simulink library "PowerFlowLib2013amdl"  (Simulink 8.1)
settings: Solver=ode45  StartTime=0.0  StopTime=10.0  RelTol=1e-3
undefined symbols (not defined in the file or in its folder): AirProp, C, F1, Fanmap, Fld1, Fld2, fueltankdata, HydProp, HydraulicLoad, IBFD_exc, L, LoadFluidProps, magnitude, MSSN, n_alghts, PumpProp, pwr_alghts, R_fd_exc, Rcore, Ts, VBFD_exc
libraries: PowerFlowLib x32, simulink x14, powerlib_extras x2, dspstat3 x2
(part 9 of 11)

== system PowerFlowLib2013amdl/Energy & Power Systems/Electrical/Battery/BATTERY/SOC  ==
  INITIAL SOC : Inport
  DCHG CT : Inport  Port=2
  CHG CT : Inport  Port=3
  CHG_DCHG_SIGNAL : Inport  Port=4
  Add1 : Sum  Inputs=+-
  Memory1 : Memory  X0=INITIAL_SOC
  Multiport Switch1 : MultiPortSwitch  DiagnosticForDefault=None
  SOC _ DISCHARGE : Subsystem
  SOC_CHARGE : Subsystem
  Saturation : Saturate  UpperLimit=1  LowerLimit=0
  DYNAMIC SOC : Outport
  NET DCHG CURRENT : Outport  Port=2
  wires:
  Saturation/1 -> Memory1/1, DYNAMIC SOC/1
  Memory1/1 -> Multiport Switch1/4
  Add1/1 -> SOC_CHARGE/2(NET BTRY CT), SOC _ DISCHARGE/2(NET BTRY CT), NET DCHG CURRENT/1
  INITIAL SOC/1 -> SOC_CHARGE/1(INITIAL SOC), SOC _ DISCHARGE/1(INTIAL SOC)
  Multiport Switch1/1 -> Saturation/1
  SOC_CHARGE/1(DYNAMIC SOC) -> Multiport Switch1/3
  DCHG CT/1 -> Add1/1
  CHG CT/1 -> Add1/2
  CHG_DCHG_SIGNAL/1 -> Multiport Switch1/1
  SOC _ DISCHARGE/1(DYNAMIC SOC) -> Multiport Switch1/2

== system PowerFlowLib2013amdl/Energy & Power Systems/Electrical/Converters/Chopper (Averaged)/duty ratio ==
  d(t) : Inport
  Fcn : Fcn  Expr=1-u
  d1(t) : Outport
  d2(t) : Outport  Port=2
  wires:
  d(t)/1 -> d1(t)/1, Fcn/1
  Fcn/1 -> d2(t)/1

== system PowerFlowLib2013amdl/Energy & Power Systems/Electrical/Inverters/ inverter/Three-Phase Full Bridge Inverter CONSTANT FREQUENCY1 ==
  Vdc : Inport
  Inverter current : Inport  Port=2
  Add : Sum
  Constant : Constant  Value=Tr
  Constant1 : Constant  Value=Tf
  Constant2 : Constant  Value=Fsw
  Constant3 : Constant  Value=VCEsat
  No. of IGBT switches : Gain  Gain=Nsw
  "No. of series vol drops " : Gain  Gain=3
  Product : Product  RndMeth=Zero
  Switch Loss : Subsystem
  Total Loss : Outport
  Switching Loss : Outport  Port=2
  Conduction Loss : Outport  Port=3
  wires:
  Constant/1 -> Switch Loss/2(Trise)
  Constant1/1 -> Switch Loss/3(Tfall)
  Inverter current/1 -> Switch Loss/4(Inverter phase current), Product/1
  Switch Loss/1(Switch Loss) -> No. of IGBT switches/1
  Constant2/1 -> Switch Loss/5(Fsw mean)
  Vdc/1 -> Switch Loss/1(Vdc)
  Constant3/1 -> "No. of series vol drops "/1
  "No. of series vol drops "/1 -> Product/2
  Add/1 -> Total Loss/1
  No. of IGBT switches/1 -> Add/1, Switching Loss/1
  Product/1 -> Add/2, Conduction Loss/1

== system PowerFlowLib2013amdl/Energy & Power Systems/Electrical/Inverters/1phs Inverter (2-level) - average/Dot Product ==
  In1 : Inport
  In2 : Inport  Port=2
  S-Function : S-Function  FunctionName=sdotproduct  EnableBusSupport=off
  Out1 : Outport
  wires:
  S-Function/1 -> Out1/1
  In1/1 -> S-Function/1
  In2/1 -> S-Function/2

== system PowerFlowLib2013amdl/Energy & Power Systems/Electrical/Inverters/1phs Inverter (2-level) - average/Dot Product1 ==
  In1 : Inport
  In2 : Inport  Port=2
  S-Function : S-Function  FunctionName=sdotproduct  EnableBusSupport=off
  Out1 : Outport
  wires:
  S-Function/1 -> Out1/1
  In1/1 -> S-Function/1
  In2/1 -> S-Function/2

== system PowerFlowLib2013amdl/Energy & Power Systems/Electrical/Inverters/1phs Inverter (2-level) - switching/2-level PWM ==
  d(t) : Inport
  Data Type Conversion : DataTypeConversion  SaturateOnIntegerOverflow=on  RndMeth=Zero
  Data Type Conversion1 : DataTypeConversion  SaturateOnIntegerOverflow=on  RndMeth=Zero
  Relational Operator : RelationalOperator  Operator=<=  InputSameDT=on
  Relational Operator1 : RelationalOperator  InputSameDT=on
  Tri(t) : Subsystem  mask(Repeating table){rep_seq_t=[0 1/f_s/2 1/f_s], rep_seq_y=[0 1 0]}
      mask prompts: rep_seq_t "Time values:"; rep_seq_y "Output values:"
      mask help: Output a repeating sequence of numbers specified in a table of time-value pairs. Values of time should be monotonically increasing.
      mask init:
      | if (length(rep_seq_t) ~= length(rep_seq_y)),
      |   error('Length of time vector and output vector must be the same.')
      | end
      | dbl_rep_seq_t = double(rep_seq_t);
      | dbl_rep_seq_y = double(rep_seq_y);
      | period = max(dbl_rep_seq_t) - min(dbl_rep_seq_t);
      | period = str2num(sprintf('%0.5g',period));
      | s = round(length(dbl_rep_seq_t)/50);
      | if s > 0
      |   pts = [1:s:length(dbl_rep_seq_t)];
      |   L   = length(pts);
      | else
      |   L   = length(dbl_rep_seq_t);
      |   pts = [1:L];
      | end
      | 
      | disp_seq_t = reshape(dbl_rep_seq_t(pts),L,1);
      | disp_seq_y = reshape(dbl_rep_seq_y(pts),L,1);
      | disp_period = max(disp_seq_t) - min(disp_seq_t);
      | 
      | disp_seq_t  = repmat(disp_seq_t,1,3) + (ones(L,1)*(disp_period*[0,1,2]));
      | disp_seq_t = [ disp_seq_t(:); disp_seq_t(end) ];
      | disp_seq_y = repmat(disp_seq_y,1,3);
      | disp_seq_y = [ disp_seq_y(:); disp_seq_y(1) ];
      mask Help: Repeats cycle given in table. Time values should be monotonically increasing.
      mask Display: plot( disp_seq_t, disp_seq_y )
  q1(t) : Outport
  q2(t) : Outport  Port=2
  wires:
  Relational Operator/1 -> Data Type Conversion/1
  Tri(t)/1(Out1) -> Relational Operator/1, Relational Operator1/1
  Relational Operator1/1 -> Data Type Conversion1/1
  d(t)/1 -> Relational Operator/2, Relational Operator1/2
  Data Type Conversion/1 -> q1(t)/1
  Data Type Conversion1/1 -> q2(t)/1

== system PowerFlowLib2013amdl/Energy & Power Systems/Electrical/Inverters/1phs Inverter (2-level) - switching/Dot Product ==
  In1 : Inport
  In2 : Inport  Port=2
  S-Function : S-Function  FunctionName=sdotproduct  EnableBusSupport=off
  Out1 : Outport
  wires:
  S-Function/1 -> Out1/1
  In1/1 -> S-Function/1
  In2/1 -> S-Function/2

== system PowerFlowLib2013amdl/Energy & Power Systems/Electrical/Inverters/1phs Inverter (2-level) - switching/Dot Product1 ==
  In1 : Inport
  In2 : Inport  Port=2
  S-Function : S-Function  FunctionName=sdotproduct  EnableBusSupport=off
  Out1 : Outport
  wires:
  S-Function/1 -> Out1/1
  In1/1 -> S-Function/1
  In2/1 -> S-Function/2

== system PowerFlowLib2013amdl/Energy & Power Systems/Electrical/Inverters/Inverter (Average)/abc 2 dq ==
  I/P 3 phase : Inport
  angle : Inport  Port=2
  Constant : Constant  Value=2*pi/3
  Constant1 : Constant  Value=2*pi/3
  Demux2 : Demux  Outputs=3
  Gain1 : Gain  Gain=-2/3
  Gain2 : Gain  Gain=2/3
  Mux : Mux  Inputs=2
  Product{,1..5} (6 alike) : Product  RndMeth=Zero
  Sum : Sum  Inputs=|+-
  Sum1 : Sum  Inputs=|+++
  Sum2 : Sum  Inputs=|++
  Sum3 : Sum  Inputs=|+++
  Trigonometric Function : Trigonometry
  Trigonometric Function1 : Trigonometry  Operator=cos
  Trigonometric Function2 : Trigonometry
  Trigonometric Function3 : Trigonometry  Operator=cos
  Trigonometric Function4 : Trigonometry
  Trigonometric Function5 : Trigonometry  Operator=cos
  "O/P 2 phase " : Outport
  wires:
  angle/1 -> Trigonometric Function1/1, Trigonometric Function/1, Sum/1, Sum2/1
  I/P 3 phase/1 -> Demux2/1
  Mux/1 -> "O/P 2 phase "/1
  Trigonometric Function1/1 -> Product2/1
  Demux2/1 -> Product2/2, Product/2
  Constant/1 -> Sum/2
  Constant1/1 -> Sum2/2
  Sum/1 -> Trigonometric Function2/1, Trigonometric Function3/1
  Sum2/1 -> Trigonometric Function4/1, Trigonometric Function5/1
  Demux2/2 -> Product3/2, Product4/2
  Trigonometric Function3/1 -> Product3/1
  Trigonometric Function5/1 -> Product1/1
  Demux2/3 -> Product1/2, Product5/2
  Product2/1 -> Sum1/1
  Product3/1 -> Sum1/2
  Product1/1 -> Sum1/3
  Sum1/1 -> Gain2/1
  Gain2/1 -> Mux/1
  Trigonometric Function/1 -> Product/1
  Trigonometric Function2/1 -> Product4/1
  Trigonometric Function4/1 -> Product5/1
  Product/1 -> Sum3/1
  Product4/1 -> Sum3/2
  Product5/1 -> Sum3/3
  Sum3/1 -> Gain1/1
  Gain1/1 -> Mux/2

== system PowerFlowLib2013amdl/Energy & Power Systems/Electrical/Loads/Constant Current Load/abc to qd0 ==
  note: abc to qd0 reference frame transform (using
      | Krause's notation q = direct axis, d = quadrature axis)
  V_a : Inport
  V_b : Inport  Port=2
  V_c : Inport  Port=3
  Fcn : Fcn  Expr=2/3*(u[1]*cos(0)+u[2]*cos(-2*pi/3)+u[3]*cos(2*pi/3))
  Fcn1 : Fcn  Expr=2/3*(u[1]*sin(0)+u[2]*sin(-2*pi/3)+u[3]*sin(2*pi/3))
  Fcn2 : Fcn  Expr=1/3*(u[1]+u[2]+u[3])
  Mux : Mux  Inputs=3
  V_q : Outport  InitialOutput=0
  V_d : Outport  Port=2  InitialOutput=0
  V_o : Outport  Port=3  InitialOutput=0
  wires:
  Fcn/1 -> V_q/1
  Fcn1/1 -> V_d/1
  Mux/1 -> Fcn/1, Fcn1/1, Fcn2/1
  V_c/1 -> Mux/3
  V_b/1 -> Mux/2
  V_a/1 -> Mux/1
  Fcn2/1 -> V_o/1

== system PowerFlowLib2013amdl/Energy & Power Systems/Electrical/Loads/Constant Power Load/abc to qd0 ==
  note: abc to qd0 reference frame transform (using
      | Krause's notation q = direct axis, d = quadrature axis)
  V_a : Inport
  V_b : Inport  Port=2
  V_c : Inport  Port=3
  Fcn : Fcn  Expr=2/3*(u[1]*cos(0)+u[2]*cos(-2*pi/3)+u[3]*cos(2*pi/3))
  Fcn1 : Fcn  Expr=2/3*(u[1]*sin(0)+u[2]*sin(-2*pi/3)+u[3]*sin(2*pi/3))
  Fcn2 : Fcn  Expr=1/3*(u[1]+u[2]+u[3])
  Mux : Mux  Inputs=3
  V_q : Outport  InitialOutput=0
  V_d : Outport  Port=2  InitialOutput=0
  V_o : Outport  Port=3  InitialOutput=0
  wires:
  Fcn/1 -> V_q/1
  Fcn1/1 -> V_d/1
  Mux/1 -> Fcn/1, Fcn1/1, Fcn2/1
  V_c/1 -> Mux/3
  V_b/1 -> Mux/2
  V_a/1 -> Mux/1
  Fcn2/1 -> V_o/1

== system PowerFlowLib2013amdl/Energy & Power Systems/Electrical/Loads/Enabled_AC_Loadloss/Enabled Subsystem ==
  "Vdq0 " : Inport
  CURRENT BASED LOADS : Subsystem
  IMPEDANCE BASED LOADS : Subsystem
  POWER BASED LOADS : Subsystem
  Sum of Elements : Sum  Inputs=+++
  Idq0 : Outport
  loss : Outport  Port=2
  wires:
  "Vdq0 "/1 -> IMPEDANCE BASED LOADS/1(Vdq0), POWER BASED LOADS/1(Vdq0)
  POWER BASED LOADS/1(Idq0) -> Sum of Elements/1
  CURRENT BASED LOADS/1(Idqo) -> Sum of Elements/2
  Sum of Elements/1 -> Idq0/1
  IMPEDANCE BASED LOADS/1(Idq0) -> Sum of Elements/3
  POWER BASED LOADS/2(loss) -> loss/1

== system PowerFlowLib2013amdl/Energy & Power Systems/Electrical/Loads/Enabled_AC_Loadloss/Enabled Subsystem1 ==
  "Vdq0 " : Inport
  Ext vector : Inport  Port=2
  CURRENT BASED LOADS : Subsystem
  Demux : Demux  Outputs=3
  POWER BASED LOADS : Subsystem
  Sum of Elements : Sum
  Idq0 : Outport
  wires:
  CURRENT BASED LOADS/1(Idqo) -> Sum of Elements/2
  POWER BASED LOADS/1(Idq0) -> Sum of Elements/1
  Sum of Elements/1 -> Idq0/1
  Ext vector/1 -> Demux/1
  "Vdq0 "/1 -> POWER BASED LOADS/1(Vdq0)
  Demux/1 -> POWER BASED LOADS/2(P)
  Demux/2 -> POWER BASED LOADS/3(Q)
  Demux/3 -> CURRENT BASED LOADS/1(Iconst RMS)

== system PowerFlowLib2013amdl/Energy & Power Systems/Electrical/Loss Estimation/Three-Phase ACTIVE RECTIFIER/Switch Loss ==
  Vdc : Inport
  Trise : Inport  Port=2
  Tfall : Inport  Port=3
  Inverter Phae current : Inport  Port=4
  Fsw mean : Inport  Port=5
  Add : Sum
  Divide : Product  Inputs=****
  Gain : Gain  Gain=0.5
  Switching Loss : Outport
  wires:
  Gain/1 -> Divide/2
  Vdc/1 -> Divide/1
  Trise/1 -> Add/1
  Tfall/1 -> Add/2
  Add/1 -> Gain/1
  Inverter Phae current/1 -> Divide/3
  Fsw mean/1 -> Divide/4
  Divide/1 -> Switching Loss/1

== system PowerFlowLib2013amdl/Energy & Power Systems/Electrical/Loss Estimation/Three-Phase ACTIVE RECTIFIER/Switching Frequency ==
  Vdc : Inport
  Source Vol (RMS) : Inport  Port=2
  H-Band : Inport  Port=3
  Lls : Inport  Port=4
  theta : Inport  Port=5
  Add : Sum  Inputs=+-
  Divide : Product  Inputs=**
  Divide1 : Product  Inputs=*/
  Divide2 : Product  Inputs=***
  Gain : Gain  Gain=sqrt(2)
  Gain1 : Gain  Gain=1/(2*pi)
  Gain2 : Gain  Gain=4
  Math Function : Math  Operator=square  SaturateOnIntegerOverflow=on
  Math Function1 : Math  Operator=square  SaturateOnIntegerOverflow=on
  Mean : dspstat3/Mean  run=on  reset_popup=None  InputProcessing=Columns as channels (frame based)  directionMode=Each column  dimension=1  treatSBRowAsCol=on  roiEnable=off  roiType=Rectangles  roiPortion=Entire ROI  roiOutput=Individual statistics for each ROI  roiFlag=off  outputDataTypeStr=Inherit: Same as accumulator  outputLastDataTypeStr=Inherit: Same as accumulator  outputMin=[]  outputMax=[]  roundingMode=Floor  overflowMode=off
  Scope8 : Scope  NumInputPorts=4
      settings: TimeRange=1  YMin=313.1~98040~-1~-5  YMax=313.35~98180~1~5  SaveName=ScopeData9
  Sine : simulink/Lookup Tables/Sine  Formula=sin(2*pi*u)  NumDataPoints=(2^5)+1  OutputWordLength=16
  Zero-Order Hold : ZeroOrderHold  SampleTime=Ts
  Inst. fsw : Outport
  Mean fsw : Outport  Port=2
  wires:
  Vdc/1 -> Divide2/3, Math Function/1, Scope8/1
  Source Vol (RMS)/1 -> Gain/1
  theta/1 -> Gain1/1
  Gain/1 -> Divide/1
  Math Function/1 -> Add/1
  Divide/1 -> Math Function1/1
  Sine/1 -> Divide/2
  Gain1/1 -> Sine/1
  Math Function1/1 -> Add/2
  Add/1 -> Divide1/1, Scope8/2
  H-Band/1 -> Gain2/1
  Gain2/1 -> Divide2/1
  Lls/1 -> Divide2/2
  Divide2/1 -> Divide1/2, Scope8/4
  Divide1/1 -> Zero-Order Hold/1, Inst. fsw/1, Scope8/3
  Mean/1 -> Mean fsw/1
  Zero-Order Hold/1 -> Mean/1

== system PowerFlowLib2013amdl/Energy & Power Systems/Electrical/Loss Estimation/Three-Phase Full Bridge Inverter CONSTANT FREQUENCY/Switch Loss ==
  Vdc : Inport
  Trise : Inport  Port=2
  Tfall : Inport  Port=3
  Inverter phase current : Inport  Port=4
  Fsw mean : Inport  Port=5
  Add : Sum
  Divide : Product  Inputs=****
  Gain : Gain  Gain=0.5
  Switch Loss : Outport
  wires:
  Vdc/1 -> Divide/1
  Trise/1 -> Add/1
  Tfall/1 -> Add/2
  Add/1 -> Gain/1
  Inverter phase current/1 -> Divide/3
  Fsw mean/1 -> Divide/4
  Divide/1 -> Switch Loss/1
  Gain/1 -> Divide/2

== system PowerFlowLib2013amdl/Energy & Power Systems/Electrical/Loss Estimation/Three-Phase Full Bridge Inverter VARIABLE FREQUENCY/Switch Loss ==
  Vdc : Inport
  Trise : Inport  Port=2
  Tfall : Inport  Port=3
  Inverter Phae current : Inport  Port=4
  Fsw mean : Inport  Port=5
  Add : Sum
  Divide : Product  Inputs=****
  Gain : Gain  Gain=0.5
  Switching Loss : Outport
  wires:
  Divide/1 -> Switching Loss/1
  Fsw mean/1 -> Divide/4
  Inverter Phae current/1 -> Divide/3
  Add/1 -> Gain/1
  Tfall/1 -> Add/2
  Trise/1 -> Add/1
  Vdc/1 -> Divide/1
  Gain/1 -> Divide/2

== system PowerFlowLib2013amdl/Energy & Power Systems/Electrical/Loss Estimation/Three-Phase Full Bridge Inverter VARIABLE FREQUENCY/Switching Frequency ==
  Vdc : Inport
  Machine vol (RMS) : Inport  Port=2
  H-Band : Inport  Port=3
  Lls : Inport  Port=4
  theta : Inport  Port=5
  Add : Sum  Inputs=+-
  Divide : Product  Inputs=**
  Divide1 : Product  Inputs=*/
  Divide2 : Product  Inputs=***
  Gain : Gain  Gain=sqrt(2)
  Gain1 : Gain  Gain=1/(2*pi)
  Gain2 : Gain  Gain=4
  Math Function : Math  Operator=square  SaturateOnIntegerOverflow=on
  Math Function1 : Math  Operator=square  SaturateOnIntegerOverflow=on
  Mean : dspstat3/Mean  run=on  reset_popup=None  InputProcessing=Columns as channels (frame based)  directionMode=Each column  dimension=1  treatSBRowAsCol=on  roiEnable=off  roiType=Rectangles  roiPortion=Entire ROI  roiOutput=Individual statistics for each ROI  roiFlag=off  outputDataTypeStr=Inherit: Same as accumulator  outputLastDataTypeStr=Inherit: Same as accumulator  outputMin=[]  outputMax=[]  roundingMode=Floor  overflowMode=off
  Scope8 : Scope  NumInputPorts=4
      settings: TimeRange=1  YMin=313.1~98040~-1~-5  YMax=313.35~98180~1~5  SaveName=ScopeData9
  Sine : simulink/Lookup Tables/Sine  Formula=sin(2*pi*u)  NumDataPoints=(2^5)+1  OutputWordLength=16
  Zero-Order Hold : ZeroOrderHold  SampleTime=Ts
  Inst. fsw : Outport
  Mean fsw : Outport  Port=2
  wires:
  Zero-Order Hold/1 -> Mean/1
  Mean/1 -> Mean fsw/1
  Divide1/1 -> Scope8/3, Inst. fsw/1, Zero-Order Hold/1
  Divide2/1 -> Scope8/4, Divide1/2
  Lls/1 -> Divide2/2
  Gain2/1 -> Divide2/1
  H-Band/1 -> Gain2/1
  Add/1 -> Scope8/2, Divide1/1
  Math Function1/1 -> Add/2
  Gain1/1 -> Sine/1
  Sine/1 -> Divide/2
  Divide/1 -> Math Function1/1
  Math Function/1 -> Add/1
  Gain/1 -> Divide/1
  theta/1 -> Gain1/1
  Machine vol (RMS)/1 -> Gain/1
  Vdc/1 -> Scope8/1, Math Function/1, Divide2/3

== system PowerFlowLib2013amdl/Energy & Power Systems/Electrical/Machines/Induction motor/D-axis block ==
  vds : Inport
  wr*pqr : Inport  Port=2
  Integrator : Integrator
  Integrator1 : Integrator
  Mux : Mux  Inputs=3
  Mux1 : Mux  Inputs=3
  Mux2 : Mux  Inputs=2
  Mux3 : Mux  Inputs=2
  i_ds : Fcn  Expr=1/IM_Xls*(u[2]-u[1])
  pmd : Fcn  Expr=IM_XM*(u[1]/IM_Xls+u[2]/IM_Xplr)
  psi_dr : Fcn  Expr=IM_wb*(-u[2]/IM_wb+IM_rrp/IM_Xplr*(u[1]-u[3]))
  psi_ds : Fcn  Expr=IM_wb*(u[2]+IM_rs/IM_Xls*(u[3]-u[1]))
  pds : Outport
  ids : Outport  Port=2
  pdr : Outport  Port=3
  wires:
  i_ds/1 -> ids/1
  Mux3/1 -> i_ds/1
  wr*pqr/1 -> Mux1/2
  Integrator1/1 -> pdr/1, Mux2/2, Mux1/3
  Integrator/1 -> pds/1, Mux3/2, Mux2/1, Mux/1
  psi_dr/1 -> Integrator1/1
  psi_ds/1 -> Integrator/1
  Mux2/1 -> pmd/1
  Mux1/1 -> psi_dr/1
  pmd/1 -> Mux1/1, Mux3/1, Mux/3
  Mux/1 -> psi_ds/1
  vds/1 -> Mux/2

== system PowerFlowLib2013amdl/Energy & Power Systems/Electrical/Machines/Induction motor/Power Loss Measurement ==
  vqd0s : Inport
  iqd0s : Inport  Port=2
  T_em : Inport  Port=3
  wr_mech : Inport  Port=4
  Gain1 : Gain  Gain=1/Rcore
  Gain2 : Gain  Gain=[3/2 3/2 1]
  Gain3 : Gain  Gain=IM_rs
  Gain4 : Gain  Gain=[3/2 3/2 1].^2
  Gain5 : Gain  Gain=[3/2 3/2 1].^2
  Math Function : Math  Operator=square  SaturateOnIntegerOverflow=on
  Math Function1 : Math  Operator=square  SaturateOnIntegerOverflow=on
  Product : Product  RndMeth=Zero
  Product1 : Product  RndMeth=Zero
  Sum : Sum  Inputs=+
  Sum1 : Sum  Inputs=+-|
  Sum2 : Sum  Inputs=+
  Sum4 : Sum  Inputs=+
  Sum5 : Sum
  P_el : Outport
  P_m : Outport  Port=2
  P_loss : Outport  Port=3
  P_el_loss : Outport  Port=4
  wires:
  Product/1 -> Gain2/1
  vqd0s/1 -> Product/1, Math Function/1
  iqd0s/1 -> Product/2, Math Function1/1
  Gain2/1 -> Sum/1
  Sum/1 -> P_el/1, Sum1/1
  Product1/1 -> P_m/1, Sum1/2
  T_em/1 -> Product1/1
  wr_mech/1 -> Product1/2
  Sum1/1 -> P_loss/1
  Gain1/1 -> Gain5/1
  Gain3/1 -> Gain4/1
  Math Function/1 -> Gain1/1
  Math Function1/1 -> Gain3/1
  Sum2/1 -> Sum5/1
  Sum4/1 -> Sum5/2
  Sum5/1 -> P_el_loss/1
  Gain4/1 -> Sum4/1  "Copper Losses"
  Gain5/1 -> Sum2/1  "Core Loss"

== system PowerFlowLib2013amdl/Energy & Power Systems/Electrical/Machines/Induction motor/Q-axis block ==
  vqs : Inport
  wr*pdr : Inport  Port=2
  Integrator : Integrator
  Integrator1 : Integrator
  Mux : Mux  Inputs=3
  Mux1 : Mux  Inputs=3
  Mux2 : Mux  Inputs=2
  Mux3 : Mux  Inputs=2
  i_qs : Fcn  Expr=1/IM_Xls*(u[2]-u[1])
  pmq : Fcn  Expr=IM_XM*(u[1]/IM_Xls+u[2]/IM_Xplr)
  psi_qr : Fcn  Expr=IM_wb*(u[2]/IM_wb+IM_rrp/IM_Xplr*(u[1]-u[3]))
  psi_qs : Fcn  Expr=IM_wb*(u[2]+IM_rs/IM_Xls*(u[3]-u[1]))
  pqs : Outport
  iqs : Outport  Port=2
  pqr : Outport  Port=3
  wires:
  i_qs/1 -> iqs/1
  Mux3/1 -> i_qs/1
  wr*pdr/1 -> Mux1/2
  Integrator1/1 -> pqr/1, Mux2/2, Mux1/3
  Integrator/1 -> pqs/1, Mux3/2, Mux2/1, Mux/1
  psi_qr/1 -> Integrator1/1
  psi_qs/1 -> Integrator/1
  Mux2/1 -> pmq/1
  Mux1/1 -> psi_qr/1
  pmq/1 -> Mux1/1, Mux3/1, Mux/3
  Mux/1 -> psi_qs/1
  vqs/1 -> Mux/2

== system PowerFlowLib2013amdl/Energy & Power Systems/Electrical/Machines/Permanent Magnet Synchronous Generator1/Generator Power Loss1 ==
  Ploss : Inport
  Tamb : Inport  Port=2
  Gain1 : Gain  Gain=1/mc_exciter
  Heat Trasnfer : Subsystem
  Integrator : Integrator  InitialConditionSource=external
  Sum : Sum  Inputs=|+-
  Ts : Outport
  Pdiss : Outport  Port=2
  wires:
  Gain1/1 -> Integrator/1
  Heat Trasnfer/1(Pdiss) -> Pdiss/1, Sum/2
  Ploss/1 -> Sum/1
  Sum/1 -> Gain1/1
  Integrator/1 -> Heat Trasnfer/2(Ts), Ts/1
  Tamb/1 -> Heat Trasnfer/1(Tamb), Integrator/2

== system PowerFlowLib2013amdl/Energy & Power Systems/Electrical/Machines/Permanent Magnet Synchronous Generator1/Power Loss Measurement ==
  vqd0s : Inport
  iqd0s : Inport  Port=2
  T_em : Inport  Port=3
  wr_mech : Inport  Port=4
  Gain1 : Gain  Gain=1e-10
  Gain2 : Gain  Gain=[3/2 3/2 1]
  Gain3 : Gain  Gain=Rs_pm
  Gain4 : Gain  Gain=[3/2 3/2 1].^2
  Gain5 : Gain  Gain=[3/2 3/2 1].^2
  Math Function : Math  Operator=square  SaturateOnIntegerOverflow=on
  Math Function1 : Math  Operator=square  SaturateOnIntegerOverflow=on
  Product : Product  RndMeth=Zero
  Product1 : Product  RndMeth=Zero
  Sum : Sum  Inputs=+
  Sum1 : Sum  Inputs=-+|
  Sum2 : Sum  Inputs=+
  Sum4 : Sum  Inputs=+
  Sum5 : Sum
  P_el : Outport
  P_m : Outport  Port=2
  P_loss : Outport  Port=3
  P_el_loss : Outport  Port=4
  wires:
  Product/1 -> Gain2/1
  vqd0s/1 -> Product/1, Math Function/1
  iqd0s/1 -> Product/2, Math Function1/1
  Gain2/1 -> Sum/1
  Sum/1 -> P_el/1, Sum1/1
  Product1/1 -> P_m/1, Sum1/2
  T_em/1 -> Product1/1
  wr_mech/1 -> Product1/2
  Sum1/1 -> P_loss/1
  Gain1/1 -> Gain5/1
  Gain3/1 -> Gain4/1
  Math Function/1 -> Gain1/1
  Math Function1/1 -> Gain3/1
  Sum2/1 -> Sum5/1
  Sum4/1 -> Sum5/2
  Sum5/1 -> P_el_loss/1
  Gain4/1 -> Sum4/1  "Copper Losses"
  Gain5/1 -> Sum2/1  "Core Loss"

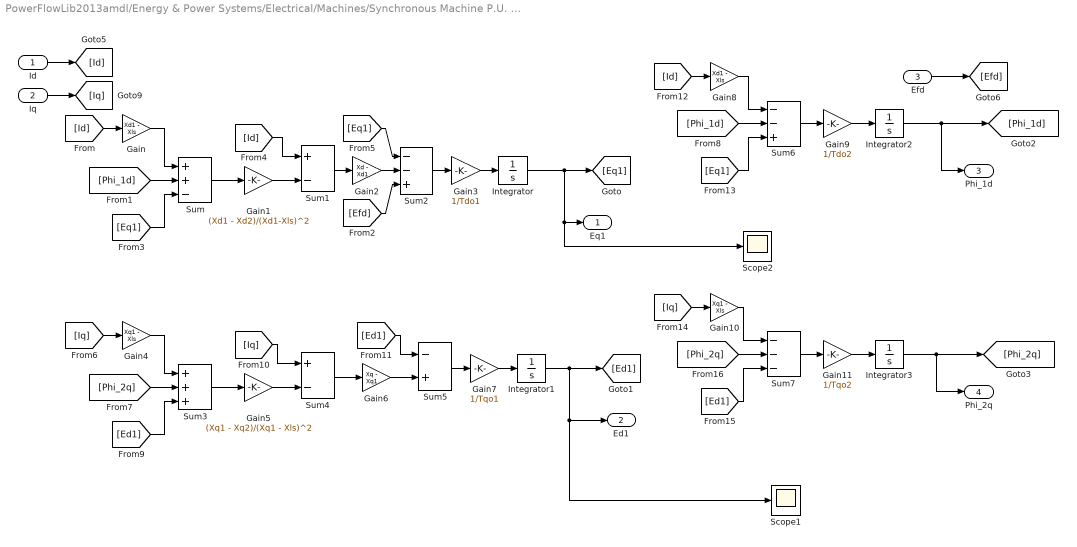
== system PowerFlowLib2013amdl/Energy & Power Systems/Electrical/Machines/Synchronous Machine P.U. dq0/Dynamics ==
  Id : Inport
  Iq : Inport  Port=2
  Efd : Inport  Port=3
  Gain : Gain  Gain=Xd1 - Xls
  Gain1 : Gain  Gain=(Xd1 - Xd2)/(Xd1-Xls)^2
  Gain10 : Gain  Gain=Xq1 - Xls
  Gain11 : Gain  Gain=1/Tqo2
  Gain2 : Gain  Gain=Xd - Xd1
  Gain3 : Gain  Gain=1/Tdo1
  Gain4 : Gain  Gain=Xq1 - Xls
  Gain5 : Gain  Gain=(Xq1 - Xq2)/(Xq1 - Xls)^2
  Gain6 : Gain  Gain=Xq - Xq1
  Gain7 : Gain  Gain=1/Tqo1
  Gain8 : Gain  Gain=Xd1 - Xls
  Gain9 : Gain  Gain=1/Tdo2
  Integrator{,1..3} (4 alike) : Integrator
  Scope1 : Scope
      settings: SaveName=ScopeData6
  Scope2 : Scope
      settings: SaveName=ScopeData7
  Sum : Sum  Inputs=++-
  Sum1 : Sum  Inputs=+-
  Sum2 : Sum  Inputs=--+
  Sum3 : Sum  Inputs=+++
  Sum4 : Sum  Inputs=+-
  Sum5 : Sum  Inputs=-+
  Sum6 : Sum  Inputs=--+
  Sum7 : Sum  Inputs=---
  Eq1 : Outport
  Ed1 : Outport  Port=2
  Phi_1d : Outport  Port=3
  Phi_2q : Outport  Port=4
  wires:
  Efd/1 -> [Efd]
  Iq/1 -> [Iq]
  Id/1 -> [Id]
  Integrator3/1 -> Phi_2q/1, [Phi_2q]
  Gain11/1 -> Integrator3/1
  Sum7/1 -> Gain11/1
  [Ed1] -> Sum7/3
  [Phi_2q] -> Sum7/2
  Gain10/1 -> Sum7/1
  [Iq] -> Gain10/1
  Integrator2/1 -> Phi_1d/1, [Phi_1d]
  Gain9/1 -> Integrator2/1
  Sum6/1 -> Gain9/1
  [Eq1] -> Sum6/3
  [Phi_1d] -> Sum6/2
  Gain8/1 -> Sum6/1
  [Id] -> Gain8/1
  Gain7/1 -> Integrator1/1
  Sum5/1 -> Gain7/1
  Gain6/1 -> Sum5/2
  [Ed1] -> Sum5/1
  Sum4/1 -> Gain6/1
  Gain5/1 -> Sum4/2
  [Iq] -> Sum4/1
  Sum3/1 -> Gain5/1
  [Ed1] -> Sum3/3
  [Phi_2q] -> Sum3/2
  Gain4/1 -> Sum3/1
  [Iq] -> Gain4/1
  Integrator1/1 -> Scope1/1, Ed1/1, [Ed1]
  Gain3/1 -> Integrator/1
  Sum2/1 -> Gain3/1
  [Efd] -> Sum2/3
  Gain2/1 -> Sum2/2
  [Eq1] -> Sum2/1
  Sum1/1 -> Gain2/1
  Gain1/1 -> Sum1/2
  [Id] -> Sum1/1
  Sum/1 -> Gain1/1
  [Eq1] -> Sum/3
  [Phi_1d] -> Sum/2
  Gain/1 -> Sum/1
  [Id] -> Gain/1
  Integrator/1 -> Scope2/1, Eq1/1, [Eq1]

== system PowerFlowLib2013amdl/Energy & Power Systems/Electrical/Machines/Synchronous Machine P.U. dq0/Electromagnetic Torque Output Power ==
  note: Torque from Damper Windings
  note: Torque from Field Winding
  Id : Inport
  Iq : Inport  Port=2
  Eq1 : Inport  Port=3
  Ed1 : Inport  Port=4
  Phi_1d : Inport  Port=5
  Phi_2q : Inport  Port=6
  Gain : Gain  Gain=(Xd2 - Xls)/(Xd1 - Xls)
  Gain1 : Gain  Gain=(Xq2 - Xls)/(Xq1 - Xls)
  Gain2 : Gain  Gain=(Xd1 - Xd2)/(Xd1-Xls)
  Gain3 : Gain  Gain=(Xq1 - Xq2)/(Xq1-Xls)
  Gain4 : Gain  Gain=(Xq2 - Xd2)
  Product{,1..4} (5 alike) : Product  RndMeth=Zero
  Sum : Sum
  Sum1 : Sum  Inputs=+-+
  Sum2 : Sum
  TE : Outport
  wires:
  Sum2/1 -> TE/1
  Sum1/1 -> Sum2/2
  Sum/1 -> Sum2/1
  Gain1/1 -> Sum/2
  Gain/1 -> Sum/1
  Gain4/1 -> Sum1/3
  Gain2/1 -> Sum1/1
  Gain3/1 -> Sum1/2
  Product4/1 -> Gain4/1
  [Iq] -> Product4/2
  [Id] -> Product4/1
  Product3/1 -> Gain3/1
  [Phi_2q] -> Product3/2
  [Id] -> Product3/1
  Product2/1 -> Gain2/1
  [Phi_1d] -> Product2/2
  [Iq] -> Product2/1
  Product1/1 -> Gain1/1
  [Id] -> Product1/2
  [Ed1] -> Product1/1
  Product/1 -> Gain/1
  [Iq] -> Product/2
  [Eq1] -> Product/1
  Iq/1 -> [Iq]
  Phi_2q/1 -> [Phi_2q]
  Phi_1d/1 -> [Phi_1d]
  Ed1/1 -> [Ed1]
  Eq1/1 -> [Eq1]
  Id/1 -> [Id]

== system PowerFlowLib2013amdl/Energy & Power Systems/Electrical/Machines/Synchronous Machine P.U. dq0/Generator Power Loss ==
  Ed : Inport
  Eq : Inport  Port=2
  Id : Inport  Port=3
  Iq : Inport  Port=4
  Te : Inport  Port=5
  w/ws : Inport  Port=6
  Bus Creator : BusCreator  Inputs=6
  Gain1 : Gain  Gain=SB
  Gain2 : Gain  Gain=SB
  Gain3 : Gain  Gain=SB
  Product : Product  RndMeth=Zero
  Product1 : Product  RndMeth=Zero
  Product2 : Product  RndMeth=Zero
  Sum1 : Sum  Inputs=-+
  Sum2 : Sum
  PE : Outport
  PM : Outport  Port=2
  PLOSS : Outport  Port=3
  m : Outport  Port=4
  wires:
  Gain3/1 -> PM/1
  Gain1/1 -> PE/1
  Gain2/1 -> PLOSS/1
  Bus Creator/1 -> m/1
  [nu] -> Bus Creator/6  "nu"
  [Te] -> Bus Creator/5  "Te"
  [Iq] -> Bus Creator/4  "Iq"
  [Eq] -> Bus Creator/3  "Vq"
  [Id] -> Bus Creator/2  "Id"
  [Ed] -> Bus Creator/1  "Vd"
  Sum1/1 -> Gain2/1
  Product2/1 -> Gain3/1, Sum1/2
  Sum2/1 -> Gain1/1, Sum1/1
  Product1/1 -> Sum2/2
  Product/1 -> Sum2/1
  [nu] -> Product2/2
  [Te] -> Product2/1
  [Iq] -> Product1/2
  [Eq] -> Product1/1
  [Id] -> Product/2
  [Ed] -> Product/1
  w/ws/1 -> [nu]
  Te/1 -> [Te]
  Iq/1 -> [Iq]
  Id/1 -> [Id]
  Eq/1 -> [Eq]
  Ed/1 -> [Ed]

== system PowerFlowLib2013amdl/Energy & Power Systems/Electrical/Machines/Synchronous Machine P.U. dq0/Generator Power Loss1 ==
  Ploss : Inport
  Tamb : Inport  Port=2
  Gain1 : Gain  Gain=1/mc_gen
  Heat Trasnfer : Subsystem
  Integrator : Integrator  InitialConditionSource=external
  Sum : Sum  Inputs=|+-
  Ts : Outport
  Pdiss : Outport  Port=2
  wires:
  Gain1/1 -> Integrator/1
  Heat Trasnfer/1(Pdiss) -> Pdiss/1, Sum/2
  Ploss/1 -> Sum/1
  Sum/1 -> Gain1/1
  Integrator/1 -> Heat Trasnfer/2(Ts), Ts/1
  Tamb/1 -> Heat Trasnfer/1(Tamb), Integrator/2

== system PowerFlowLib2013amdl/Energy & Power Systems/Electrical/Machines/Synchronous Machine P.U. dq0/Stator Voltage ==
  Id : Inport
  Iq : Inport  Port=2
  Eq1 : Inport  Port=3
  Ed1 : Inport  Port=4
  Phi_1d : Inport  Port=5
  Phi_2q : Inport  Port=6
  w/ws : Inport  Port=7
  Gain : Gain  Gain=(Xq2 - Xls)/(Xq1 - Xls)
  Gain1 : Gain  Gain=(Xq1 - Xq2)/(Xq1 - Xls)
  Gain2 : Gain  Gain=(Xq2 - Xd2)
  Gain3 : Gain  Gain=(Xd2 - Xls)/(Xd1 - Xls)
  Gain4 : Gain  Gain=(Xd1 - Xd2)/(Xd1 - Xls)
  Gain5 : Gain  Gain=Rs
  Gain6 : Gain  Gain=Xd2+XTL
  Gain7 : Gain  Gain=Rs+RTL
  Gain8 : Gain  Gain=Xd2+XTL
  Product{,1..3} (4 alike) : Product  RndMeth=Zero
  Sum : Sum
  Sum1 : Sum  Inputs=+-+
  Sum2 : Sum  Inputs=--+
  Sum3 : Sum  Inputs=-++
  Ed : Outport
  Eq : Outport  Port=2
  wires:
  Gain7/1 -> Sum2/2
  Product3/1 -> Sum2/1
  Sum2/1 -> Eq/1  "Vq"
  Sum3/1 -> Ed/1  "Vd"
  Product2/1 -> Sum3/3
  Gain2/1 -> Sum1/3
  Product1/1 -> Sum3/2
  Gain8/1 -> Product3/1
  Gain5/1 -> Sum3/1
  Gain6/1 -> Product2/2
  Id/1 -> Gain8/1, Gain5/1
  Product/1 -> Sum2/3
  w/ws/1 -> Product2/1, Product3/2, Product/2, Product1/2
  Sum1/1 -> Product1/1
  Sum/1 -> Product/1
  Gain1/1 -> Sum1/2
  Gain/1 -> Sum1/1
  Gain3/1 -> Sum/1
  Gain4/1 -> Sum/2
  Phi_1d/1 -> Gain4/1
  Eq1/1 -> Gain3/1
  Iq/1 -> Gain2/1, Gain7/1, Gain6/1
  Phi_2q/1 -> Gain1/1
  Ed1/1 -> Gain/1

== system PowerFlowLib2013amdl/Energy & Power Systems/Electrical/Systems/Generation Unit Sync-Sync/Chopper (Averaged) ==
  vin : Inport
  q : Inport  Port=2
  1/R : Gain  Gain=1/(R_fd_exc*VBFD_exc/IBFD_exc)/100/2*3/100  SaturateOnIntegerOverflow=on  OutDataTypeStr=Inherit: Same as input  ParamDataTypeStr=Inherit: Same as input
  Dot Product : DotProduct  InputSameDT=on  OutDataTypeStr=Inherit: Inherit via internal rule
  Dot Product1 : DotProduct  InputSameDT=on  OutDataTypeStr=Inherit: Inherit via internal rule
  Gain2 : Gain  Gain=1000*2/3
  Saturation : Saturate  UpperLimit=1  LowerLimit=0
  iout : Outport
  iin : Outport  Port=2
  wires:
  Dot Product1/1 -> iin/1
  Saturation/1 -> Dot Product1/2, Dot Product/2
  1/R/1 -> Gain2/1
  Dot Product/1 -> 1/R/1
  q/1 -> Saturation/1
  vin/1 -> Dot Product/1
  Gain2/1 -> Dot Product1/1, iout/1

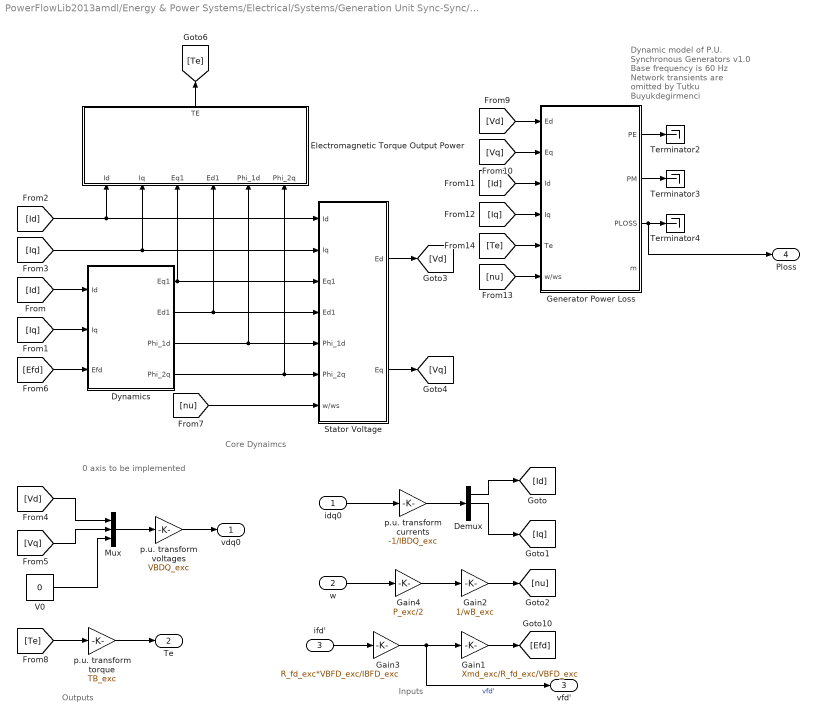
== system PowerFlowLib2013amdl/Energy & Power Systems/Electrical/Systems/Generation Unit Sync-Sync/Exciter ==
  note: 0 axis to be implemented
  note: Inputs
  note: Outputs
  note: Core Dynaimcs
  note: Dynamic model of P.U. Synchronous Generators v1.0
      | Base frequency is 60 Hz
      | Network transients are omitted
      | by Tutku Buyukdegirmenci
  idq0 : Inport
  w : Inport  Port=2
  ifd' : Inport  Port=3
  Demux : Demux  Outputs=3
  Dynamics : Subsystem
  Electromagnetic Torque Output Power : Subsystem
  Gain1 : Gain  Gain=Xmd_exc/R_fd_exc/VBFD_exc
  Gain2 : Gain  Gain=1/wB_exc
  Gain3 : Gain  Gain=R_fd_exc*VBFD_exc/IBFD_exc
  Gain4 : Gain  Gain=P_exc/2
  Generator Power Loss : Subsystem
  Mux : Mux  Inputs=3
  Stator Voltage : Subsystem
  Terminator2 : Terminator
  Terminator3 : Terminator
  Terminator4 : Terminator
  V0 : Constant  Value=0
  p.u. transform currents : Gain  Gain=-1/IBDQ_exc
  p.u. transform torque : Gain  Gain=TB_exc
  p.u. transform voltages : Gain  Gain=VBDQ_exc
  vdq0 : Outport
  Te : Outport  Port=2
  vfd' : Outport  Port=3
  Ploss : Outport  Port=4
  wires:
  Dynamics/1(Eq1) -> Stator Voltage/3(Eq1), Electromagnetic Torque Output Power/3(Eq1)
  Dynamics/2(Ed1) -> Stator Voltage/4(Ed1), Electromagnetic Torque Output Power/4(Ed1)
  Dynamics/3(Phi_1d) -> Stator Voltage/5(Phi_1d), Electromagnetic Torque Output Power/5(Phi_1d)
  Dynamics/4(Phi_2q) -> Stator Voltage/6(Phi_2q), Electromagnetic Torque Output Power/6(Phi_2q)
  Stator Voltage/2(Eq) -> [Vq]
  Stator Voltage/1(Ed) -> [Vd]
  w/1 -> Gain4/1
  Demux/1 -> [Id]
  Demux/2 -> [Iq]
  Gain2/1 -> [nu]
  [Id] -> Dynamics/1(Id)
  [Iq] -> Dynamics/2(Iq)
  [Id] -> Stator Voltage/1(Id), Electromagnetic Torque Output Power/1(Id)
  [Iq] -> Stator Voltage/2(Iq), Electromagnetic Torque Output Power/2(Iq)
  Mux/1 -> p.u. transform voltages/1
  [Vd] -> Mux/1
  [Vq] -> Mux/2
  V0/1 -> Mux/3
  [nu] -> Stator Voltage/7(w/ws)
  Electromagnetic Torque Output Power/1(TE) -> [Te]
  [Te] -> p.u. transform torque/1
  p.u. transform currents/1 -> Demux/1
  p.u. transform torque/1 -> Te/1
  [Vd] -> Generator Power Loss/1(Ed)
  [Vq] -> Generator Power Loss/2(Eq)
  [Id] -> Generator Power Loss/3(Id)
  [Iq] -> Generator Power Loss/4(Iq)
  [nu] -> Generator Power Loss/6(w/ws)
  [Te] -> Generator Power Loss/5(Te)
  Generator Power Loss/1(PE) -> Terminator2/1
  Generator Power Loss/2(PM) -> Terminator3/1
  Generator Power Loss/3(PLOSS) -> Ploss/1, Terminator4/1
  p.u. transform voltages/1 -> vdq0/1
  idq0/1 -> p.u. transform currents/1
  ifd'/1 -> Gain3/1
  Gain1/1 -> [Efd]
  Gain3/1 -> vfd'/1, Gain1/1  "vfd'"
  [Efd] -> Dynamics/3(Efd)
  Gain4/1 -> Gain2/1

== system PowerFlowLib2013amdl/Energy & Power Systems/Electrical/Systems/Generation Unit Sync-Sync/Generator ==
  note: Dynamic model of P.U. Synchronous Generators v1.0
      | Base frequency is 60 Hz
      | Network transients are omitted
      | by Tutku Buyukdegirmenci
  note: Core Dynaimcs
  note: Outputs
  note: Inputs
  note: 0 axis to be implemented
  idq0 : Inport
  w : Inport  Port=2
  ifd' : Inport  Port=3
  Demux : Demux  Outputs=3
  Dynamics : Subsystem
  Electromagnetic Torque Output Power : Subsystem
  Gain1 : Gain  Gain=Xmd/R_fd/VBFD
  Gain2 : Gain  Gain=1/wB
  Gain3 : Gain  Gain=R_fd*VBFD/IBFD
  Gain4 : Gain  Gain=P/2
  Generator Power Loss : Subsystem
  Mux : Mux  Inputs=3
  Stator Voltage : Subsystem
  Terminator2 : Terminator
  Terminator3 : Terminator
  Terminator4 : Terminator
  V0 : Constant  Value=0
  p.u. transform currents : Gain  Gain=-1/IBDQ
  p.u. transform torque : Gain  Gain=TB
  p.u. transform voltages : Gain  Gain=VBDQ
  vdq0 : Outport
  Te : Outport  Port=2
  vfd' : Outport  Port=3
  Ploss : Outport  Port=4
  wires:
  Gain4/1 -> Gain2/1
  [Efd] -> Dynamics/3(Efd)
  Gain3/1 -> vfd'/1, Gain1/1  "vfd'"
  Gain1/1 -> [Efd]
  ifd'/1 -> Gain3/1
  idq0/1 -> p.u. transform currents/1
  p.u. transform voltages/1 -> vdq0/1
  Generator Power Loss/3(PLOSS) -> Ploss/1, Terminator4/1
  Generator Power Loss/2(PM) -> Terminator3/1
  Generator Power Loss/1(PE) -> Terminator2/1
  [Te] -> Generator Power Loss/5(Te)
  [nu] -> Generator Power Loss/6(w/ws)
  [Iq] -> Generator Power Loss/4(Iq)
  [Id] -> Generator Power Loss/3(Id)
  [Vq] -> Generator Power Loss/2(Eq)
  [Vd] -> Generator Power Loss/1(Ed)
  p.u. transform torque/1 -> Te/1
  p.u. transform currents/1 -> Demux/1
  [Te] -> p.u. transform torque/1
  Electromagnetic Torque Output Power/1(TE) -> [Te]
  [nu] -> Stator Voltage/7(w/ws)
  V0/1 -> Mux/3
  [Vq] -> Mux/2
  [Vd] -> Mux/1
  Mux/1 -> p.u. transform voltages/1
  [Iq] -> Electromagnetic Torque Output Power/2(Iq), Stator Voltage/2(Iq)
  [Id] -> Electromagnetic Torque Output Power/1(Id), Stator Voltage/1(Id)
  [Iq] -> Dynamics/2(Iq)
  [Id] -> Dynamics/1(Id)
  Gain2/1 -> [nu]
  Demux/2 -> [Iq]
  Demux/1 -> [Id]
  w/1 -> Gain4/1
  Stator Voltage/1(Ed) -> [Vd]
  Stator Voltage/2(Eq) -> [Vq]
  Dynamics/4(Phi_2q) -> Electromagnetic Torque Output Power/6(Phi_2q), Stator Voltage/6(Phi_2q)
  Dynamics/3(Phi_1d) -> Electromagnetic Torque Output Power/5(Phi_1d), Stator Voltage/5(Phi_1d)
  Dynamics/2(Ed1) -> Electromagnetic Torque Output Power/4(Ed1), Stator Voltage/4(Ed1)
  Dynamics/1(Eq1) -> Electromagnetic Torque Output Power/3(Eq1), Stator Voltage/3(Eq1)

== system PowerFlowLib2013amdl/Energy & Power Systems/Electrical/Systems/Generator Bus/Compare To Constant ==
  u : Inport
  Compare : RelationalOperator  Operator===  OutDataTypeStr=fixdt(0, 8)  InputSameDT=on
  Constant : Constant  DisableCoverage=on  Value=const  OutDataTypeStr=Inherit: Inherit via back propagation
  y : Outport
  wires:
  u/1 -> Compare/1
  Constant/1 -> Compare/2
  Compare/1 -> y/1

== system PowerFlowLib2013amdl/Energy & Power Systems/Electrical/Systems/Generator Bus/Compare To Constant1 ==
  u : Inport
  Compare : RelationalOperator  Operator===  OutDataTypeStr=fixdt(0, 8)  InputSameDT=on
  Constant : Constant  DisableCoverage=on  Value=const  OutDataTypeStr=Inherit: Inherit via back propagation
  y : Outport
  wires:
  u/1 -> Compare/1
  Constant/1 -> Compare/2
  Compare/1 -> y/1

== system PowerFlowLib2013amdl/Energy & Power Systems/Electrical/Systems/Generator Bus/Compare To Constant2 ==
  u : Inport
  Compare : RelationalOperator  Operator===  OutDataTypeStr=fixdt(0, 8)  InputSameDT=on
  Constant : Constant  DisableCoverage=on  Value=const  OutDataTypeStr=Inherit: Inherit via back propagation
  y : Outport
  wires:
  u/1 -> Compare/1
  Constant/1 -> Compare/2
  Compare/1 -> y/1

== system PowerFlowLib2013amdl/Energy & Power Systems/Electrical/Systems/Generator Bus/Compare To Constant3 ==
  u : Inport
  Compare : RelationalOperator  Operator===  OutDataTypeStr=fixdt(0, 8)  InputSameDT=on
  Constant : Constant  DisableCoverage=on  Value=const  OutDataTypeStr=Inherit: Inherit via back propagation
  y : Outport
  wires:
  u/1 -> Compare/1
  Constant/1 -> Compare/2
  Compare/1 -> y/1

== system PowerFlowLib2013amdl/Energy & Power Systems/Electrical/Systems/three-phase  full-bridge  inverter/Three-Phase Full Bridge Inverter CONSTANT FREQUENCY1 ==
  Vdc : Inport
  Inverter current : Inport  Port=2
  Add : Sum
  Constant : Constant  Value=Tr
  Constant1 : Constant  Value=Tf
  Constant2 : Constant  Value=Fsw
  Constant3 : Constant  Value=VCEsat
  Display : Display
  No. of IGBT switches : Gain  Gain=Nsw
  "No. of series vol drops " : Gain  Gain=3
  Product : Product  RndMeth=Zero
  Switch Loss : Subsystem
  Total Loss : Outport
  Switching Loss : Outport  Port=2
  Conduction Loss : Outport  Port=3
  wires:
  Product/1 -> Conduction Loss/1, Add/2
  No. of IGBT switches/1 -> Switching Loss/1, Add/1
  Add/1 -> Total Loss/1
  "No. of series vol drops "/1 -> Product/2
  Constant3/1 -> "No. of series vol drops "/1
  Vdc/1 -> Switch Loss/1(Vdc)
  Constant2/1 -> Switch Loss/5(Fsw mean)
  Switch Loss/1(Switch Loss) -> No. of IGBT switches/1
  Inverter current/1 -> Product/1, Switch Loss/4(Inverter phase current)
  Constant1/1 -> Switch Loss/3(Tfall)
  Constant/1 -> Switch Loss/2(Trise)

== system PowerFlowLib2013amdl/Energy & Power Systems/Thermal/ECS/Air-Air HX/Air_properties_in_flows_hot_and_cold ==
  In_flow_bus_hot : Inport
  In_flow_bus_cold : Inport  Port=2
  Bus Creator : BusCreator  Inputs=5
  Bus Creator3 : BusCreator  Inputs=5
  air_properties_in_cold : Subsystem
  air_properties_in_hot : Subsystem
  air_properties_in_hot1 : Outport
  air_properties_in_cold1 : Outport  Port=2
  wires:
  air_properties_in_hot/4(K_air_Wm-1K-2) -> Bus Creator/4  "K_air"
  air_properties_in_cold/5(Pr) -> Bus Creator3/5  "Pr"
  air_properties_in_hot/5(Pr) -> Bus Creator/5  "Pr"
  In_flow_bus_cold/1 -> air_properties_in_cold/1(In_flow_bus_cold)
  In_flow_bus_hot/1 -> air_properties_in_hot/1(In_flow_bus_hot)
  Bus Creator/1 -> air_properties_in_hot1/1
  Bus Creator3/1 -> air_properties_in_cold1/1
  air_properties_in_hot/3(mu_air_Pa.s) -> Bus Creator/3  "mu_air"
  air_properties_in_hot/2(cp_air_Jkg-1K-1) -> Bus Creator/2  "cp_air"
  air_properties_in_hot/1(rho_air_kgm-3) -> Bus Creator/1  "rho_air"
  air_properties_in_cold/4(K_air_Wm-1K-2) -> Bus Creator3/4  "K_air"
  air_properties_in_cold/3(mu_air_Pa.s) -> Bus Creator3/3  "mu_air"
  air_properties_in_cold/2(cp_air_Jkg-1K-1) -> Bus Creator3/2  "cp_air"
  air_properties_in_cold/1(rho_air_kgm-3) -> Bus Creator3/1  "rho_air"

== system PowerFlowLib2013amdl/Energy & Power Systems/Thermal/ECS/Air-Air HX/C_T_c_av ==
  In_flow_bus : Inport
  air_properties : Inport  Port=2
  Tot_thermal_resist : Inport  Port=3
  Add : Sum
  Bus Selector : BusSelector  OutputSignals=mdot_kgps
  Bus Selector1 : BusSelector  OutputSignals=cp_air
  Constant : Constant
  Divide : Product  Inputs=***
  Divide1 : Product  Inputs=*/
  Gain : Gain  Gain=2
  C_T_c_av : Outport
  wires:
  Divide1/1 -> C_T_c_av/1
  Add/1 -> Divide1/2
  Constant/1 -> Add/2
  Gain/1 -> Divide1/1, Add/1
  Divide/1 -> Gain/1
  Bus Selector1/1 -> Divide/3  "<cp_air>"
  Bus Selector/1 -> Divide/2  "<mdot_kgps>"
  Tot_thermal_resist/1 -> Divide/1  "R_tot_c"
  In_flow_bus/1 -> Bus Selector/1
  air_properties/1 -> Bus Selector1/1

== system PowerFlowLib2013amdl/Energy & Power Systems/Thermal/ECS/Air-Air HX/C_T_c_i ==
  In_flow_bus : Inport
  air_properties : Inport  Port=2
  Tot_thermal_resist : Inport  Port=3
  HX_parameters : Inport  Port=4
  Add : Sum
  Bus Selector : BusSelector  OutputSignals=mdot_kgps
  Bus Selector1 : BusSelector  OutputSignals=cp_air
  Bus Selector2 : BusSelector  OutputSignals=m_cm,cp_hx
  Constant : Constant
  Divide : Product  Inputs=***
  Divide2 : Product  Inputs=**///
  Gain : Gain  Gain=2
  Gain1 : Gain  Gain=2
  C_T_c_i : Outport
  wires:
  In_flow_bus/1 -> Bus Selector/1
  air_properties/1 -> Bus Selector1/1
  Tot_thermal_resist/1 -> Divide/1  "R_tot"
  Bus Selector/1 -> Divide/2, Divide2/1  "<mdot_kgps>"
  Bus Selector1/1 -> Divide/3, Divide2/2  "<cp_air>"
  Divide/1 -> Gain/1
  Gain/1 -> Add/1
  Constant/1 -> Add/2
  HX_parameters/1 -> Bus Selector2/1
  Bus Selector2/1 -> Divide2/3  "<m_cm>"
  Bus Selector2/2 -> Divide2/4  "<cp_hx>"
  Add/1 -> Divide2/5
  Gain1/1 -> C_T_c_i/1
  Divide2/1 -> Gain1/1

== system PowerFlowLib2013amdl/Energy & Power Systems/Thermal/ECS/Air-Air HX/C_T_h_av ==
  In_flow_bus : Inport
  air_properties : Inport  Port=2
  Tot_thermal_resist : Inport  Port=3
  Add : Sum
  Bus Selector : BusSelector  OutputSignals=mdot_kgps
  Bus Selector1 : BusSelector  OutputSignals=cp_air
  Constant : Constant
  Divide : Product  Inputs=***
  Divide1 : Product  Inputs=*/
  Gain : Gain  Gain=2
  C_T_h_av : Outport
  wires:
  Divide1/1 -> C_T_h_av/1
  Add/1 -> Divide1/2
  Constant/1 -> Add/2
  Gain/1 -> Divide1/1, Add/1
  Divide/1 -> Gain/1
  Bus Selector1/1 -> Divide/3  "<cp_air>"
  Bus Selector/1 -> Divide/2  "<mdot_kgps>"
  Tot_thermal_resist/1 -> Divide/1  "R_tot_h"
  In_flow_bus/1 -> Bus Selector/1
  air_properties/1 -> Bus Selector1/1

== system PowerFlowLib2013amdl/Energy & Power Systems/Thermal/ECS/Air-Air HX/C_T_h_i ==
  In_flow_bus : Inport
  air_properties : Inport  Port=2
  Tot_thermal_resist : Inport  Port=3
  HX_parameters : Inport  Port=4
  Add : Sum
  Bus Selector : BusSelector  OutputSignals=mdot_kgps
  Bus Selector1 : BusSelector  OutputSignals=cp_air
  Bus Selector2 : BusSelector  OutputSignals=m_cm,cp_hx
  Constant : Constant
  Divide : Product  Inputs=***
  Divide2 : Product  Inputs=**///
  Gain : Gain  Gain=2
  Gain1 : Gain  Gain=2
  C_T_h_i : Outport
  wires:
  Gain1/1 -> C_T_h_i/1
  Add/1 -> Divide2/5
  Bus Selector2/2 -> Divide2/4  "<cp_hx>"
  Bus Selector2/1 -> Divide2/3  "<m_cm>"
  HX_parameters/1 -> Bus Selector2/1
  Constant/1 -> Add/2
  Gain/1 -> Add/1
  Divide/1 -> Gain/1
  Bus Selector1/1 -> Divide/3, Divide2/2  "<cp_air>"
  Bus Selector/1 -> Divide/2, Divide2/1  "<mdot_kgps>"
  Tot_thermal_resist/1 -> Divide/1  "R_tot_h"
  air_properties/1 -> Bus Selector1/1
  In_flow_bus/1 -> Bus Selector/1
  Divide2/1 -> Gain1/1

== system PowerFlowLib2013amdl/Energy & Power Systems/Thermal/ECS/Air-Air HX/Calculating_T_c_av ==
  T_cm : Inport
  In_flow_bus : Inport  Port=2
  C_t_c_av : Inport  Port=3
  Add1 : Sum  Inputs=-+
  Add3 : Sum
  Bus Selector : BusSelector  OutputSignals=temp_C
  Divide1 : Product  Inputs=**
  T_c_av_degreC : Outport
  wires:
  T_cm/1 -> Add3/1, Add1/1  "T_cm"
  In_flow_bus/1 -> Bus Selector/1
  Bus Selector/1 -> Add1/2  "<temp_C>"
  C_t_c_av/1 -> Divide1/2
  Add1/1 -> Divide1/1  "T_c_i - T_cm"
  Divide1/1 -> Add3/2
  Add3/1 -> T_c_av_degreC/1

== system PowerFlowLib2013amdl/Energy & Power Systems/Thermal/ECS/Air-Air HX/Calculating_T_h_av ==
  T_cm : Inport
  In_flow_bus : Inport  Port=2
  C_t_h_av : Inport  Port=3
  Add1 : Sum  Inputs=-+
  Add3 : Sum
  Bus Selector : BusSelector  OutputSignals=temp_C
  Divide1 : Product  Inputs=**
  T_h_av_degreC : Outport
  wires:
  Add1/1 -> Divide1/1  "T_h_i - T_cm"
  C_t_h_av/1 -> Divide1/2
  Bus Selector/1 -> Add1/2  "<temp_C>"
  In_flow_bus/1 -> Bus Selector/1
  T_cm/1 -> Add1/1, Add3/1  "T_cm"
  Add3/1 -> T_h_av_degreC/1
  Divide1/1 -> Add3/2

== system PowerFlowLib2013amdl/Energy & Power Systems/Thermal/ECS/Air-Air HX/Calculating_core_mass_temp ==
  note: dTcm/dt
  note: Tcm
  C_T_h_i : Inport
  C_T_c_i : Inport  Port=2
  C_t_cm : Inport  Port=3
  In_flow_bus_hot : Inport  Port=4
  In_flow_bus_cold : Inport  Port=5
  Add : Sum  Inputs=++-
  Bus Selector : BusSelector  OutputSignals=temp_C
  Bus Selector1 : BusSelector  OutputSignals=temp_C
  Divide : Product  Inputs=**
  Divide1 : Product  Inputs=**
  Divide2 : Product  Inputs=**
  Integrator : Integrator  InitialCondition=T_cm_0
  Core_mass_temp_C : Outport
  wires:
  Divide1/1 -> Add/3
  C_t_cm/1 -> Divide1/2
  Integrator/1 -> Core_mass_temp_C/1, Divide1/1
  Add/1 -> Integrator/1
  Divide2/1 -> Add/2
  Divide/1 -> Add/1
  Bus Selector1/1 -> Divide2/2  "<temp_C>"
  C_T_c_i/1 -> Divide2/1
  Bus Selector/1 -> Divide/2  "<temp_C>"
  C_T_h_i/1 -> Divide/1
  In_flow_bus_cold/1 -> Bus Selector1/1
  In_flow_bus_hot/1 -> Bus Selector/1

== system PowerFlowLib2013amdl/Energy & Power Systems/Thermal/ECS/Air-Air HX/Colburn_J_factor_cold ==
  Fin_prameter_ratios : Inport
  Re : Inport  Port=2
  Add : Sum
  Bus Selector : BusSelector  OutputSignals=alpha_fin,delta_fin,gamma_fin
  Constant : Constant  Value=-0.5403
  Constant1 : Constant  Value=-0.1541
  Constant2 : Constant  Value=0.1499
  Constant3 : Constant  Value=-0.0678
  Constant4 : Constant  Value=1.34
  Constant5 : Constant  Value=0.504
  Constant6 : Constant  Value=0.456
  Constant7 : Constant  Value=-1.055
  Constant8 : Constant
  Constant9 : Constant  Value=0.1
  Divide : Product  Inputs=****
  Divide1 : Product  Inputs=****
  Divide2 : Product  Inputs=**
  Gain : Gain  Gain=0.6522
  Gain1 : Gain  Gain=5.269*10^(-5)
  Re1 : Math  Operator=pow  SaturateOnIntegerOverflow=on
  Re2 : Math  Operator=pow  SaturateOnIntegerOverflow=on
  alpha_fin : Math  Operator=pow  SaturateOnIntegerOverflow=on
  alpha_fin1 : Math  Operator=pow  SaturateOnIntegerOverflow=on
  delta_fin : Math  Operator=pow  SaturateOnIntegerOverflow=on
  delta_fin1 : Math  Operator=pow  SaturateOnIntegerOverflow=on
  gamma_fin : Math  Operator=pow  SaturateOnIntegerOverflow=on
  gamma_fin1 : Math  Operator=pow  SaturateOnIntegerOverflow=on
  gamma_fin2 : Math  Operator=pow  SaturateOnIntegerOverflow=on
  Colburn_J_factor : Outport
  wires:
  Divide2/1 -> Colburn_J_factor/1
  Gain/1 -> Divide2/1
  gamma_fin2/1 -> Divide2/2
  Constant9/1 -> gamma_fin2/2
  Add/1 -> gamma_fin2/1
  Gain1/1 -> Add/1
  Constant8/1 -> Add/2
  Divide1/1 -> Gain1/1
  gamma_fin1/1 -> Divide1/4
  delta_fin1/1 -> Divide1/3
  alpha_fin1/1 -> Divide1/2
  Re2/1 -> Divide1/1
  Divide/1 -> Gain/1
  gamma_fin/1 -> Divide/4
  delta_fin/1 -> Divide/3
  alpha_fin/1 -> Divide/2
  Re1/1 -> Divide/1
  Bus Selector/3 -> gamma_fin1/1, gamma_fin/1  "<gamma_fin>"
  Bus Selector/2 -> delta_fin1/1, delta_fin/1  "<delta_fin>"
  Bus Selector/1 -> alpha_fin1/1, alpha_fin/1  "<alpha_fin>"
  Re/1 -> Re2/1, Re1/1
  Constant7/1 -> gamma_fin1/2
  Constant6/1 -> delta_fin1/2
  Constant5/1 -> alpha_fin1/2
  Constant4/1 -> Re2/2
  Constant3/1 -> gamma_fin/2
  Constant2/1 -> delta_fin/2
  Constant1/1 -> alpha_fin/2
  Constant/1 -> Re1/2
  Fin_prameter_ratios/1 -> Bus Selector/1

== system PowerFlowLib2013amdl/Energy & Power Systems/Thermal/ECS/Air-Air HX/Colburn_J_factor_hot ==
  Fin_prameter_ratios : Inport
  Re : Inport  Port=2
  Add : Sum
  Bus Selector : BusSelector  OutputSignals=alpha_fin,delta_fin,gamma_fin
  Constant : Constant  Value=-0.5403
  Constant1 : Constant  Value=-0.1541
  Constant2 : Constant  Value=0.1499
  Constant3 : Constant  Value=-0.0678
  Constant4 : Constant  Value=1.34
  Constant5 : Constant  Value=0.504
  Constant6 : Constant  Value=0.456
  Constant7 : Constant  Value=-1.055
  Constant8 : Constant
  Constant9 : Constant  Value=0.1
  Divide : Product  Inputs=****
  Divide1 : Product  Inputs=****
  Divide2 : Product  Inputs=**
  Gain : Gain  Gain=0.6522
  Gain1 : Gain  Gain=5.269*10^(-5)
  Re1 : Math  Operator=pow  SaturateOnIntegerOverflow=on
  Re2 : Math  Operator=pow  SaturateOnIntegerOverflow=on
  alpha_fin : Math  Operator=pow  SaturateOnIntegerOverflow=on
  alpha_fin1 : Math  Operator=pow  SaturateOnIntegerOverflow=on
  delta_fin : Math  Operator=pow  SaturateOnIntegerOverflow=on
  delta_fin1 : Math  Operator=pow  SaturateOnIntegerOverflow=on
  gamma_fin : Math  Operator=pow  SaturateOnIntegerOverflow=on
  gamma_fin1 : Math  Operator=pow  SaturateOnIntegerOverflow=on
  gamma_fin2 : Math  Operator=pow  SaturateOnIntegerOverflow=on
  Colburn_J_factor : Outport
  wires:
  Fin_prameter_ratios/1 -> Bus Selector/1
  Constant/1 -> Re1/2
  Constant1/1 -> alpha_fin/2
  Constant2/1 -> delta_fin/2
  Constant3/1 -> gamma_fin/2
  Constant4/1 -> Re2/2
  Constant5/1 -> alpha_fin1/2
  Constant6/1 -> delta_fin1/2
  Constant7/1 -> gamma_fin1/2
  Re/1 -> Re1/1, Re2/1
  Bus Selector/1 -> alpha_fin/1, alpha_fin1/1  "<alpha_fin>"
  Bus Selector/2 -> delta_fin/1, delta_fin1/1  "<delta_fin>"
  Bus Selector/3 -> gamma_fin/1, gamma_fin1/1  "<gamma_fin>"
  Re1/1 -> Divide/1
  alpha_fin/1 -> Divide/2
  delta_fin/1 -> Divide/3
  gamma_fin/1 -> Divide/4
  Divide/1 -> Gain/1
  Re2/1 -> Divide1/1
  alpha_fin1/1 -> Divide1/2
  delta_fin1/1 -> Divide1/3
  gamma_fin1/1 -> Divide1/4
  Divide1/1 -> Gain1/1
  Constant8/1 -> Add/2
  Gain1/1 -> Add/1
  Add/1 -> gamma_fin2/1
  Constant9/1 -> gamma_fin2/2
  gamma_fin2/1 -> Divide2/2
  Gain/1 -> Divide2/1
  Divide2/1 -> Colburn_J_factor/1
